simulink model "lab1"  (R2023b)
settings: Solver=VariableStepAuto  StartTime=0.0  StopTime=5  RelTol=1e-3
values from neighbouring files (symbols this model uses):
  C = -7    [lab1_sim.m]
  K1 = -2.482936299    [lab1_sim.m]
  tau = 0.02575805674    [lab1_sim.m]
settings Model: Creator=j368lu  LastModifiedBy=j368lu

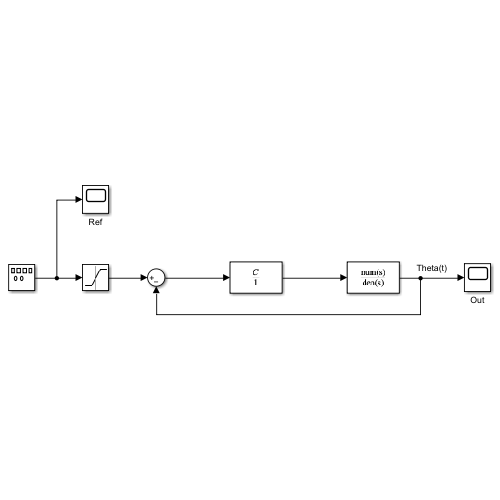
[thumbnail: Simulink's stored preview of the top-level diagram]
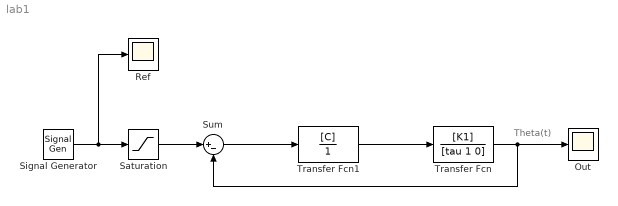
== system lab1 ==
  note: Theta(t)
  Out : Scope
  Ref : Scope
  Saturation : Saturate  UpperLimit=0.785  LowerLimit=-0.785  LinearizeAsGain=off  ZeroCross=off
  Signal Generator : SignalGenerator  WaveForm=sawtooth  Amplitude=2  Frequency=0.2
  Sum : Sum  Inputs=|+-
  Transfer Fcn : TransferFcn  Numerator=[K1]  Denominator=[tau 1 0]
  Transfer Fcn1 : TransferFcn  Numerator=[C]  Denominator=[1]
  wires:
  Transfer Fcn1/1 -> Transfer Fcn/1
  Signal Generator/1 -> Ref/1, Saturation/1
  Saturation/1 -> Sum/1
  Transfer Fcn/1 -> Out/1, Sum/2
  Sum/1 -> Transfer Fcn1/1
